simulink model "counter"  (R2020b)
settings: Solver=VariableStepAuto  StartTime=0.0  StopTime=10.0  RelTol=1e-3
settings Model: Creator=priyaD  LastModifiedBy=priyaD

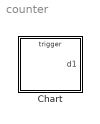
== system counter ==
  Chart : Stateflow chart  TreatAsAtomicUnit=on

== stateflow chart counter/Chart ==
  state digit1
    state one
      en: d1=1;
    state zero
      en: d1=0;
    state two
      en: d1=2;
    digit1.zero -> digit1.one : clk
    digit1.one -> digit1.two : clk
    (default) -> digit1.zero
    digit1.two -> digit1.zero : clk/{clk1}
  state digit2
    state one
      en: d1=1;
    state zero
      en: d1=0;
    state two
      en: d1=2;
    digit2.zero -> digit2.one : clk
    digit2.one -> digit2.two : clk
    (default) -> digit2.zero
    digit2.two -> digit2.zero : clk/{clk1}
  data: d1 output
  events: clk input RISING_EDGE_EVENT
